simulink model "Whiplash_IGS"  (R2021a)
settings: Solver=ode1  StartTime=0.0  StopTime=0.01  FixedStep=.001  RelTol=1e-3
undefined symbols (not defined in the file or in its folder): magnitude
settings Model: Creator=RUDRA  LastModifiedBy=RUDRA

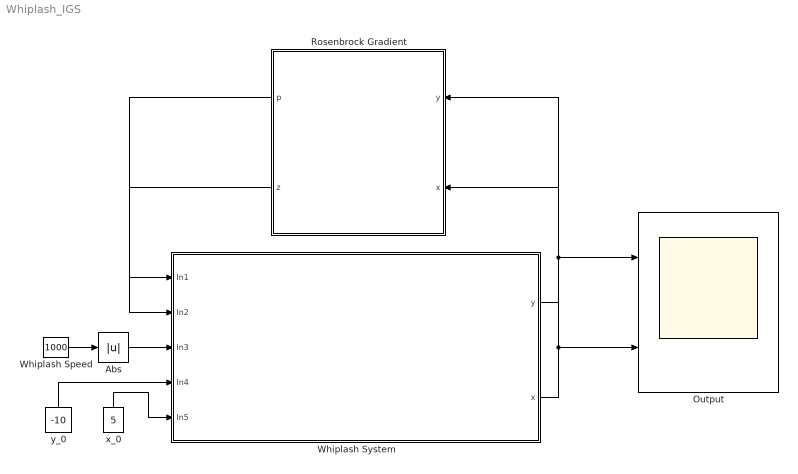
== system Whiplash_IGS ==
  Abs : Abs
  Output : Scope  NumInputPorts=2
  Rosenbrock Gradient : Subsystem
  Whiplash Speed : Constant  Value=1000  VectorParams1D=off
  Whiplash System : Subsystem
  x_0 : Constant  Value=5
  y_0 : Constant  Value=-10
  wires:
  Whiplash Speed/1 -> Abs/1
  Abs/1 -> Whiplash System/3(In3)
  y_0/1 -> Whiplash System/4(In4)
  x_0/1 -> Whiplash System/5(In5)
  Whiplash System/1(y) -> Rosenbrock Gradient/1(y), Output/1
  Whiplash System/2(x) -> Output/2, Rosenbrock Gradient/2(x)
  Rosenbrock Gradient/1(p) -> Whiplash System/1(In1)
  Rosenbrock Gradient/2(z) -> Whiplash System/2(In2)

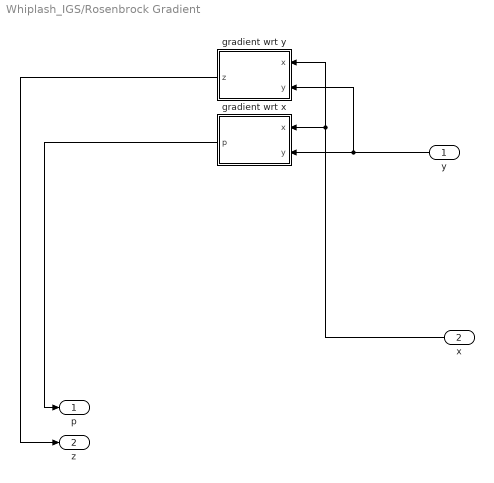
== system Whiplash_IGS/Rosenbrock Gradient ==
  y : Inport
  x : Inport  Port=2
  gradient wrt x : MATLAB Function  TreatAsAtomicUnit=on
  gradient wrt y : MATLAB Function  TreatAsAtomicUnit=on
  p : Outport
  z : Outport  Port=2
  wires:
  gradient wrt x/1(p) -> p/1
  x/1 -> gradient wrt y/1(x), gradient wrt x/1(x)
  y/1 -> gradient wrt x/2(y), gradient wrt y/2(y)
  gradient wrt y/1(z) -> z/1

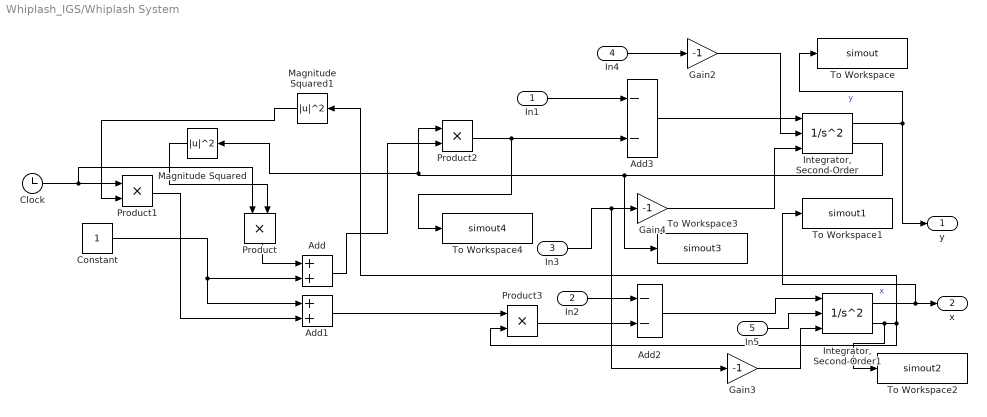
== system Whiplash_IGS/Whiplash System ==
  In1 : Inport
  In2 : Inport  Port=2
  In3 : Inport  Port=3
  In4 : Inport  Port=4
  In5 : Inport  Port=5
  Add : Sum
  Add1 : Sum
  Add2 : Sum  Inputs=--
  Add3 : Sum  Inputs=--
  Clock : Clock
  Constant : Constant
  Gain2 : Gain  Gain=-1
  Gain3 : Gain  Gain=-1
  Gain4 : Gain  Gain=-1
  "Integrator, Second-Order" : SecondOrderIntegrator  ICSourceX=external  ICX=2.0  ICSourceDXDT=external  ICDXDT=0
  "Integrator, Second-Order1" : SecondOrderIntegrator  ICSourceX=external  ICX=2.0  ICSourceDXDT=external  ICDXDT=0
  Magnitude Squared : Math  Operator=magnitude^2  SaturateOnIntegerOverflow=on
  Magnitude Squared1 : Math  Operator=magnitude^2  SaturateOnIntegerOverflow=on
  Product{,1..3} (4 alike) : Product
  To Workspace : ToWorkspace  VariableName=simout  SaveFormat=Timeseries  SampleTime=-1
  To Workspace1 : ToWorkspace  VariableName=simout1  SaveFormat=Timeseries  SampleTime=-1
  To Workspace2 : ToWorkspace  VariableName=simout2  SaveFormat=Timeseries  SampleTime=-1
  To Workspace3 : ToWorkspace  VariableName=simout3  SaveFormat=Timeseries  SampleTime=-1
  To Workspace4 : ToWorkspace  VariableName=simout4  SaveFormat=Timeseries  SampleTime=-1
  y : Outport
  x : Outport  Port=2
  wires:
  Constant/1 -> Add1/1, Add/2
  "Integrator, Second-Order"/2 -> To Workspace3/1, Magnitude Squared/1, Product2/1
  Product1/1 -> Add1/2
  "Integrator, Second-Order1"/2 -> To Workspace2/1, Magnitude Squared1/1, Product3/2
  Magnitude Squared1/1 -> Product1/2
  Clock/1 -> Product/1, Product1/1
  Product/1 -> Add/1
  Magnitude Squared/1 -> Product/2
  "Integrator, Second-Order"/1 -> y/1, To Workspace/1  "y"
  In1/1 -> Add3/1
  Add/1 -> Product2/2
  Product2/1 -> To Workspace4/1, Add3/2
  Add1/1 -> Product3/1
  Product3/1 -> Add2/2
  Add2/1 -> "Integrator, Second-Order1"/1
  In4/1 -> Gain2/1
  Gain3/1 -> "Integrator, Second-Order1"/3
  "Integrator, Second-Order1"/1 -> To Workspace1/1, x/1  "x"
  Gain4/1 -> "Integrator, Second-Order"/3
  Add3/1 -> "Integrator, Second-Order"/1
  In2/1 -> Add2/1
  In3/1 -> Gain3/1, Gain4/1
  Gain2/1 -> "Integrator, Second-Order"/2
  In5/1 -> "Integrator, Second-Order1"/2

== matlab function Whiplash_IGS/Rosenbrock Gradient/gradient wrt y ==
  data: x input; z output; y input
function z = fcn(x,y)

z = 400*(x^2+2*x-y)*(1+x)+2*x;

== matlab function Whiplash_IGS/Rosenbrock Gradient/gradient wrt x ==
  data: x input; p output; y input
function p = fcn(x,y)

p = -200*(x^2+2*x-y);
